simulink model "zad1"  (R2016a)
settings: Solver=ode4  StartTime=0.0  StopTime=10  FixedStep=0.01  RelTol=1e-3
libraries: simulink x1
settings Model: Creator=ka28161  LastModifiedBy=ka28161

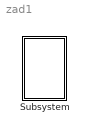
== system zad1 ==
  Subsystem : Subsystem  mask{x0=0, vx0=15, y0=5, vy0=0, M=100, G=9.81, R=2}

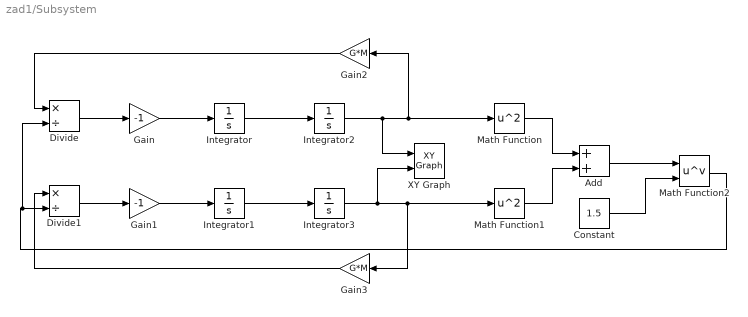
== system zad1/Subsystem ==
  Add : Sum
  Constant : Constant  Value=1.5
  Divide : Product  Inputs=*/
  Divide1 : Product  Inputs=*/
  Gain : Gain  Gain=-1
  Gain1 : Gain  Gain=-1
  Gain2 : Gain  Gain=G*M
  Gain3 : Gain  Gain=G*M
  Integrator : Integrator  InitialCondition=vx0
  Integrator1 : Integrator  InitialCondition=vy0
  Integrator2 : Integrator  InitialCondition=x0
  Integrator3 : Integrator  InitialCondition=y0
  Math Function : Math  Operator=square  SaturateOnIntegerOverflow=on
  Math Function1 : Math  Operator=square  SaturateOnIntegerOverflow=on
  Math Function2 : Math  Operator=pow  SaturateOnIntegerOverflow=on
  XY Graph : simulink/Sinks/XY Graph  xmin=-10  xmax=10  ymin=-10  ymax=10  st=-1
  wires:
  Divide1/1 -> Gain1/1
  Integrator1/1 -> Integrator3/1
  Gain1/1 -> Integrator1/1
  Gain/1 -> Integrator/1
  Integrator/1 -> Integrator2/1
  Integrator2/1 -> Gain2/1, Math Function/1, XY Graph/1
  Integrator3/1 -> Gain3/1, Math Function1/1, XY Graph/2
  Math Function1/1 -> Add/2
  Math Function/1 -> Add/1
  Math Function2/1 -> Divide/2, Divide1/2
  Constant/1 -> Math Function2/2
  Gain2/1 -> Divide/1
  Divide/1 -> Gain/1
  Add/1 -> Math Function2/1
  Gain3/1 -> Divide1/1
